simulink model "AFE_RC_OpenLoop"  (R2013b)
settings: Solver=FixedStepDiscrete  SolverMode=SingleTasking  StartTime=0.0  StopTime=5  FixedStep=Tpas  RelTol=1e-3
InitFcn:
  |  AFEsimpleparaDT1
values from neighbouring files (symbols this model uses):
  Freq = 50    [AFEsimpleparaDT1.m]
  hys = 100    [AFEsimpleparaDT1.m]
  Imax = 1.4697e+03    (= 1469.7)    [AFEsimpleparaDT1.m]
  Lac = 8.1487e-04    (= 0.00081487)    [AFEsimpleparaDT1.m]
  Tpas = 5e-5    (= 5e-05)    [AFEsimpleparaDT1.m]
  Vac = 2000    [AFEsimpleparaDT1.m]
libraries: powerlib x22, powerlib_meascontrol x7, simulink x6
settings Model: Creator=LiberT  LastModifiedBy=LiberT
settings DataIOCC: SignalLoggingSaveFormat=ModelDataLogs
settings OptimizationCC: ExpressionDepthLimit=2147483647
settings DebuggingCC: MultiTaskDSMMsg=warning  MultiTaskCondExecSysMsg=none  FcnCallInpInsideContextMsg=EnableAllAsWarning  StateNameClashWarn=warning
settings RTWCC: IncludeERTFirstTime=on

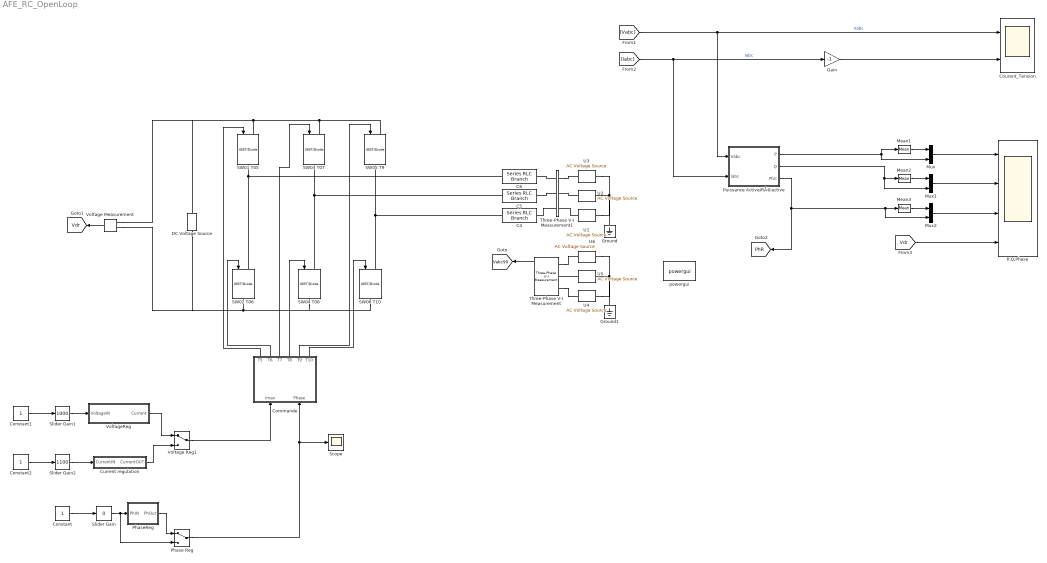
== system AFE_RC_OpenLoop ==
  C4 : powerlib/Elements/Series RLC Branch  LConnTagsString=__new0  RConnTagsString=__new0  BranchType=L  Resistance=(Vac*sqrt(2/3))^2  Inductance=Lac  SetiL0=off  InitialCurrent=0  Capacitance=300e-3  Setx0=off  InitialVoltage=0  Measurements=None
  C5 : powerlib/Elements/Series RLC Branch  LConnTagsString=__new0  RConnTagsString=__new0  BranchType=L  Resistance=(Vac*sqrt(2/3))^2  Inductance=Lac  SetiL0=off  InitialCurrent=0  Capacitance=300e-3  Setx0=off  InitialVoltage=0  Measurements=None
  C6 : powerlib/Elements/Series RLC Branch  LConnTagsString=__new0  RConnTagsString=__new0  BranchType=L  Resistance=(Vac*sqrt(2/3))^2  Inductance=Lac  SetiL0=off  InitialCurrent=0  Capacitance=300e-3  Setx0=off  InitialVoltage=0  Measurements=None
  Commande : Subsystem
  Constant : Constant
  Constant1 : Constant
  Constant2 : Constant
  Courant_Tension : Scope  NumInputPorts=2
      settings: TickLabels=on  TimeRange=0.04  YMin=-1750~-1750  YMax=1750~1750  SaveName=Courant_Tension  MaxDataPoints=50000
  Current regulation : Subsystem
  DC Voltage Source : powerlib/Electrical Sources/DC Voltage Source  Amplitude=5000  Measurements=None
  Gain : Gain  Gain=-1
  Ground : powerlib/Elements/Ground  LConnTagsString=a
  Ground1 : powerlib/Elements/Ground  LConnTagsString=a
  Mean1 : powerlib_meascontrol/Measurements/Mean  Freq=50  Vinit=0  Ts=Tpas
  Mean2 : powerlib_meascontrol/Measurements/Mean  Freq=50  Vinit=0  Ts=Tpas
  Mean3 : powerlib_meascontrol/Measurements/Mean  Freq=50  Vinit=0  Ts=Tpas
  Mux : Mux  Inputs=2
  Mux1 : Mux  Inputs=2
  Mux2 : Mux  Inputs=2
  P,Q,Phase : Scope  NumInputPorts=4
      settings: TickLabels=on  TimeRange=5  YMin=1.75e+06~-1.25e+06~-30~5000  YMax=4.5e+06~1.5e+06~25~5000  SaveName=PQ_Phi  MaxDataPoints=50000
  Phase Reg : ManualSwitch
  PhaseReg : Subsystem
  Puissance Active/RÃ©active : Subsystem
  SW01 T05 : powerlib/Power Electronics/IGBT//Diode  Ron=1e-3  Rs=1e5  Cs=Tpas  Measurements=off
  SW02 T06 : powerlib/Power Electronics/IGBT//Diode  Ron=1e-3  Rs=1e5  Cs=Tpas  Measurements=off
  SW03 T07 : powerlib/Power Electronics/IGBT//Diode  Ron=1e-3  Rs=1e5  Cs=Tpas  Measurements=off
  SW04 T08 : powerlib/Power Electronics/IGBT//Diode  Ron=1e-3  Rs=1e5  Cs=Tpas  Measurements=off
  SW05 T9 : powerlib/Power Electronics/IGBT//Diode  Ron=1e-3  Rs=1e5  Cs=Tpas  Measurements=off
  SW06 T10 : powerlib/Power Electronics/IGBT//Diode  Ron=1e-3  Rs=1e5  Cs=Tpas  Measurements=off
  Scope : Scope
      settings: YMin=-230  YMax=-160
  Slider Gain : simulink/Math Operations/Slider Gain  low=-180  gain=0  high=180
  Slider Gain1 : simulink/Math Operations/Slider Gain  low=0  gain=1000  high=5000
  Slider Gain2 : simulink/Math Operations/Slider Gain  low=500  gain=1100  high=1500
  Three-Phase V-I Measurement : powerlib/Measurements/Three-Phase V-I Measurement  VoltageMeasurement=phase-to-ground  SetLabelV=off  LabelV=Vabc  Vpu=off  VpuLL=off  CurrentMeasurement=no  SetLabelI=off  LabelI=Iabc  Ipu=off  Pbase=100e6  Vbase=500e3  OutputType=Complex  PhasorSimulation=off  PSBequivalent=0
  Three-Phase V-I Measurement1 : powerlib/Measurements/Three-Phase V-I Measurement  VoltageMeasurement=phase-to-ground  SetLabelV=on  LabelV=Vabc  Vpu=off  VpuLL=off  CurrentMeasurement=yes  SetLabelI=on  LabelI=Iabc  Ipu=off  Pbase=100e6  Vbase=500e3  OutputType=Complex  PhasorSimulation=off  PSBequivalent=0
  U1 : powerlib/Electrical Sources/AC Voltage Source  Amplitude=Vac*sqrt(2/3)  Phase=120  Frequency=Freq  SampleTime=Tpas  Measurements=Voltage
  U2 : powerlib/Electrical Sources/AC Voltage Source  Amplitude=Vac*sqrt(2/3)  Phase=-120  Frequency=Freq  SampleTime=Tpas  Measurements=Voltage
  U3 : powerlib/Electrical Sources/AC Voltage Source  Amplitude=Vac*sqrt(2/3)  Phase=0  Frequency=Freq  SampleTime=Tpas  Measurements=Voltage
  U4 : powerlib/Electrical Sources/AC Voltage Source  Amplitude=1  Phase=120-90  Frequency=Freq  SampleTime=Tpas  Measurements=Voltage
  U5 : powerlib/Electrical Sources/AC Voltage Source  Amplitude=1  Phase=-120-90  Frequency=Freq  SampleTime=Tpas  Measurements=Voltage
  U6 : powerlib/Electrical Sources/AC Voltage Source  Amplitude=1  Phase=-90  Frequency=Freq  SampleTime=Tpas  Measurements=Voltage
  Voltage Measurement : powerlib/Measurements/Voltage Measurement  PhasorSimulation=off  OutputType=Complex  PSBequivalent=0
  Voltage Reg1 : ManualSwitch
  VoltageReg : Subsystem
  powergui : powerlib/powergui  Priority=1  SimulationMode=Discrete  SolverType=Tustin  SampleTime=Tpas  frequency=50  SPID=off  DisableSnubberDevices=off  DisableRonSwitches=off  DisableVfSwitches=off  SwTol=0  Interpol=off  DisplayEquations=off  frequencyindice=50  Pbase=100e6  ErrMax=1e-4  Iterations=50  UnitsV=kV  UnitsW=MW  FunctionMessages=off  echomessages=off  HookPort=off  EnableUseOfTLC=off  x0status=blocks  RestoreLinks=warning  ResistiveCurrentMeasurement=off  Frange=[0:2:500]  Ylog=off  Xlog=on  ShowGrid=off  save=off  variable=ZData  structure=Courant_Tension  ZoomFFT=off  StartTime=0.5  cycles=225  DisplayStyle=1  fundamental=50  FreqAxis=off  MaxFrequency=500  frequencyindicesteady=1  RmsSteady=1  display=off  Ts=0  methode=off
  tag scope: PhR=global, Vabc90=global, Vdr=global
  wires:
  [Iabc] -> Gain/1, Puissance Active/RÃ©active/2(Iabc)  "Iabc"
  Commande/1(T5) -> SW01 T05/1
  Commande/2(T6) -> SW02 T06/1
  Commande/4(T8) -> SW04 T08/1
  Commande/3(T7) -> SW03 T07/1
  Commande/6(T10) -> SW06 T10/1
  Commande/5(T9) -> SW05 T9/1
  [Vabc] -> Courant_Tension/1, Puissance Active/RÃ©active/1(Vabc)  "Vabc"
  Voltage Measurement/1 -> [Vdr]
  [Vdr] -> P,Q,Phase/4
  Gain/1 -> Courant_Tension/2
  Three-Phase V-I Measurement/1 -> [Vabc90]
  Puissance Active/RÃ©active/3(PhC) -> [PhR], Mux2/2, Mean3/1
  Mux2/1 -> P,Q,Phase/3
  Puissance Active/RÃ©active/1(P) -> Mean1/1, Mux/2
  Mean1/1 -> Mux/1
  Mux/1 -> P,Q,Phase/1
  Mux1/1 -> P,Q,Phase/2
  Puissance Active/RÃ©active/2(Q) -> Mux1/2, Mean2/1
  Mean2/1 -> Mux1/1
  Mean3/1 -> Mux2/1
  Constant/1 -> Slider Gain/1
  Slider Gain/1 -> Phase Reg/2, PhaseReg/1(PhIN)
  PhaseReg/1(PhOut) -> Phase Reg/1
  Phase Reg/1 -> Commande/2(Phase), Scope/1
  Constant1/1 -> Slider Gain1/1
  Slider Gain1/1 -> VoltageReg/1(VoltageIN)
  Constant2/1 -> Slider Gain2/1
  Slider Gain2/1 -> Current regulation/1(CurrentIN)
  VoltageReg/1(Current) -> Voltage Reg1/1
  Current regulation/1(CurrentOUT) -> Voltage Reg1/2
  Voltage Reg1/1 -> Commande/1(Imax)
  connections:
  SW06 T10/RConn1 -- SW04 T08/RConn1 -- DC Voltage Source/LConn1 -- Voltage Measurement/LConn2 -- SW02 T06/RConn1
  SW01 T05/LConn1 -- DC Voltage Source/RConn1 -- Voltage Measurement/LConn1 -- SW05 T9/LConn1 -- SW03 T07/LConn1
  SW02 T06/LConn1 -- C6/LConn1 -- SW01 T05/RConn1
  SW06 T10/LConn1 -- C4/LConn1 -- SW05 T9/RConn1
  SW04 T08/LConn1 -- C5/LConn1 -- SW03 T07/RConn1
  U2/LConn1 -- U1/LConn1 -- Ground/LConn1 -- U3/LConn1
  Three-Phase V-I Measurement1/LConn1 -- C6/RConn1
  Three-Phase V-I Measurement1/RConn1 -- U3/RConn1
  U2/RConn1 -- Three-Phase V-I Measurement1/RConn2
  Three-Phase V-I Measurement1/LConn2 -- C5/RConn1
  C4/RConn1 -- Three-Phase V-I Measurement1/LConn3
  U1/RConn1 -- Three-Phase V-I Measurement1/RConn3
  U6/LConn1 -- U5/LConn1 -- U4/LConn1 -- Ground1/LConn1
  Three-Phase V-I Measurement/LConn1 -- U6/RConn1
  U5/RConn1 -- Three-Phase V-I Measurement/LConn2
  Three-Phase V-I Measurement/LConn3 -- U4/RConn1

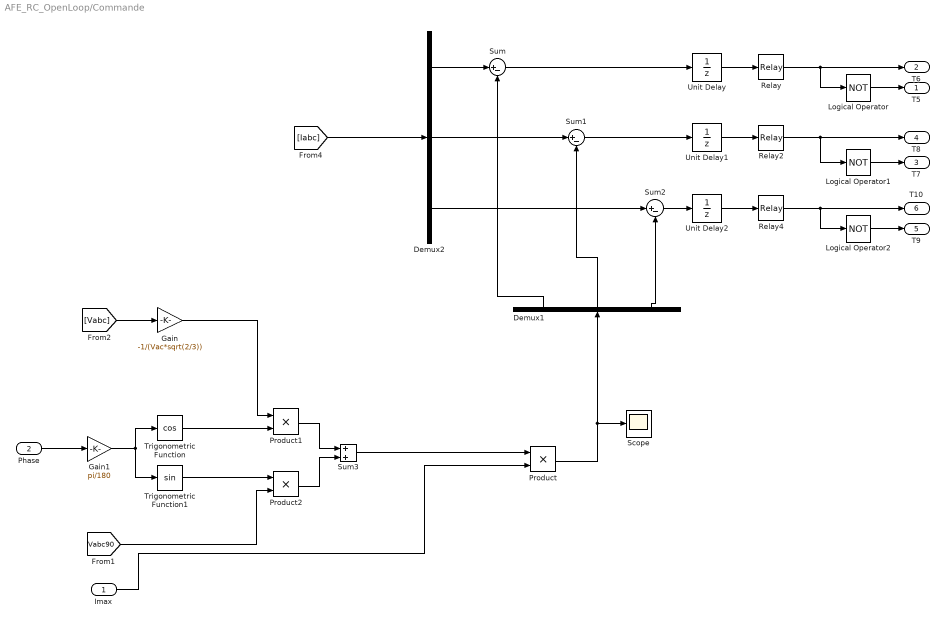
== system AFE_RC_OpenLoop/Commande ==
  Imax : Inport
  Phase : Inport  Port=2
  Demux1 : Demux  Outputs=3
  Demux2 : Demux  Outputs=3
  Gain : Gain  Gain=-1/(Vac*sqrt(2/3))
  Gain1 : Gain  Gain=pi/180
  Logical Operator : Logic  Operator=NOT  AllPortsSameDT=off
  Logical Operator1 : Logic  Operator=NOT  AllPortsSameDT=off
  Logical Operator2 : Logic  Operator=NOT  AllPortsSameDT=off
  Product : Product
  Product1 : Product
  Product2 : Product
  Relay : Relay  OnSwitchValue=hys  OffSwitchValue=-hys
  Relay2 : Relay  OnSwitchValue=hys  OffSwitchValue=-hys
  Relay4 : Relay  OnSwitchValue=hys  OffSwitchValue=-hys
  Scope : Scope
      settings: TimeRange=0.04  YMin=-1500  YMax=1500  MaxDataPoints=50000
  Sum : Sum  Inputs=|+-
  Sum1 : Sum  Inputs=|+-
  Sum2 : Sum  Inputs=|+-
  Sum3 : Sum
  Trigonometric Function : Trigonometry  Operator=cos
  Trigonometric Function1 : Trigonometry
  Unit Delay : UnitDelay  SampleTime=-1
  Unit Delay1 : UnitDelay  SampleTime=-1
  Unit Delay2 : UnitDelay  SampleTime=-1
  T5 : Outport
  T6 : Outport  Port=2
  T7 : Outport  Port=3
  T8 : Outport  Port=4
  T9 : Outport  Port=5
  T10 : Outport  Port=6
  wires:
  Demux2/1 -> Sum/1
  Demux2/2 -> Sum1/1
  Demux2/3 -> Sum2/1
  Sum/1 -> Unit Delay/1
  Sum1/1 -> Unit Delay1/1
  Sum2/1 -> Unit Delay2/1
  Unit Delay/1 -> Relay/1
  Unit Delay1/1 -> Relay2/1
  Unit Delay2/1 -> Relay4/1
  Logical Operator/1 -> T5/1
  Logical Operator1/1 -> T7/1
  Logical Operator2/1 -> T9/1
  Relay/1 -> T6/1, Logical Operator/1
  Relay2/1 -> T8/1, Logical Operator1/1
  Relay4/1 -> T10/1, Logical Operator2/1
  [Iabc] -> Demux2/1
  Demux1/2 -> Sum1/2
  Demux1/3 -> Sum2/2
  Demux1/1 -> Sum/2
  [Vabc] -> Gain/1
  Product/1 -> Scope/1, Demux1/1
  Gain/1 -> Product1/1
  Trigonometric Function/1 -> Product1/2
  [Vabc90] -> Product2/2
  Trigonometric Function1/1 -> Product2/1
  Product1/1 -> Sum3/1
  Product2/1 -> Sum3/2
  Sum3/1 -> Product/1
  Imax/1 -> Product/2
  Gain1/1 -> Trigonometric Function/1, Trigonometric Function1/1
  Phase/1 -> Gain1/1

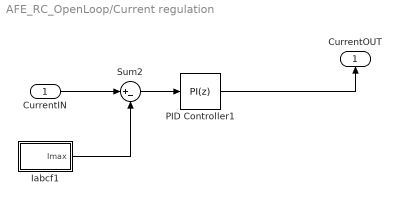
== system AFE_RC_OpenLoop/Current regulation ==
  CurrentIN : Inport
  Iabcf1 : Subsystem
  PID Controller1 : simulink/Continuous/PID Controller  Controller=PI  TimeDomain=Discrete-time  SampleTime=Tpas  IntegratorMethod=Forward Euler  FilterMethod=Forward Euler  Form=Parallel  P=5  I=0.1  D=0  N=100  InitialConditionSource=internal  InitialConditionForIntegrator=0  InitialConditionForFilter=0  ExternalReset=none  LimitOutput=on  UpperSaturationLimit=Imax  LowerSaturationLimit=0  LinearizeAsGain=on  AntiWindupMode=clamping  Kb=1  TrackingMode=off  Kt=1  PParamMin=[]  PParamMax=[]  IParamMin=[]  IParamMax=[]  DParamMin=[]  DParamMax=[]  NParamMin=[]  NParamMax=[]  KbParamMin=[]  KbParamMax=[]  KtParamMin=[]  KtParamMax=[]  POutMin=[]  POutMax=[]  IOutMin=[]  IOutMax=[]  DOutMin=[]  DOutMax=[]  NOutMin=[]  NOutMax=[]  KbOutMin=[]  KbOutMax=[]  KtOutMin=[]  KtOutMax=[]  IntegratorOutMin=[]  IntegratorOutMax=[]  FilterOutMin=[]  FilterOutMax=[]  SumOutMin=[]  SumOutMax=[]  SumI1OutMin=[]  SumI1OutMax=[]  SumI2OutMin=[]  SumI2OutMax=[]  SumI3OutMin=[]  SumI3OutMax=[]  SumDOutMin=[]  SumDOutMax=[]  SaturationOutMin=[]  SaturationOutMax=[]  IntegratorContinuousStateAttributes=''  IntegratorStateMustResolveToSignalObject=off  IntegratorRTWStateStorageClass=Auto  FilterContinuousStateAttributes=''  FilterStateMustResolveToSignalObject=off  FilterRTWStateStorageClass=Auto
  Sum2 : Sum  Inputs=|+-
  CurrentOUT : Outport
  wires:
  Iabcf1/1(Imax) -> Sum2/2
  PID Controller1/1 -> CurrentOUT/1
  Sum2/1 -> PID Controller1/1
  CurrentIN/1 -> Sum2/1

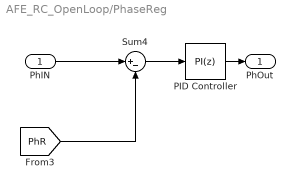
== system AFE_RC_OpenLoop/PhaseReg ==
  PhIN : Inport
  PID Controller : simulink/Continuous/PID Controller  Controller=PI  TimeDomain=Discrete-time  SampleTime=Tpas  IntegratorMethod=Forward Euler  FilterMethod=Forward Euler  Form=Parallel  P=0.48  I=8  D=0  N=100  InitialConditionSource=internal  InitialConditionForIntegrator=0  InitialConditionForFilter=0  ExternalReset=none  LimitOutput=off  UpperSaturationLimit=179.5  LowerSaturationLimit=-179.5  LinearizeAsGain=on  AntiWindupMode=clamping  Kb=1  TrackingMode=off  Kt=1  PParamMin=[]  PParamMax=[]  IParamMin=[]  IParamMax=[]  DParamMin=[]  DParamMax=[]  NParamMin=[]  NParamMax=[]  KbParamMin=[]  KbParamMax=[]  KtParamMin=[]  KtParamMax=[]  POutMin=[]  POutMax=[]  IOutMin=[]  IOutMax=[]  DOutMin=[]  DOutMax=[]  NOutMin=[]  NOutMax=[]  KbOutMin=[]  KbOutMax=[]  KtOutMin=[]  KtOutMax=[]  IntegratorOutMin=[]  IntegratorOutMax=[]  FilterOutMin=[]  FilterOutMax=[]  SumOutMin=[]  SumOutMax=[]  SumI1OutMin=[]  SumI1OutMax=[]  SumI2OutMin=[]  SumI2OutMax=[]  SumI3OutMin=[]  SumI3OutMax=[]  SumDOutMin=[]  SumDOutMax=[]  SaturationOutMin=[]  SaturationOutMax=[]  IntegratorContinuousStateAttributes=''  IntegratorStateMustResolveToSignalObject=off  IntegratorRTWStateStorageClass=Auto  FilterContinuousStateAttributes=''  FilterStateMustResolveToSignalObject=off  FilterRTWStateStorageClass=Auto
  Sum4 : Sum  Inputs=|+-
  PhOut : Outport
  wires:
  PID Controller/1 -> PhOut/1
  Sum4/1 -> PID Controller/1
  [PhR] -> Sum4/2
  PhIN/1 -> Sum4/1

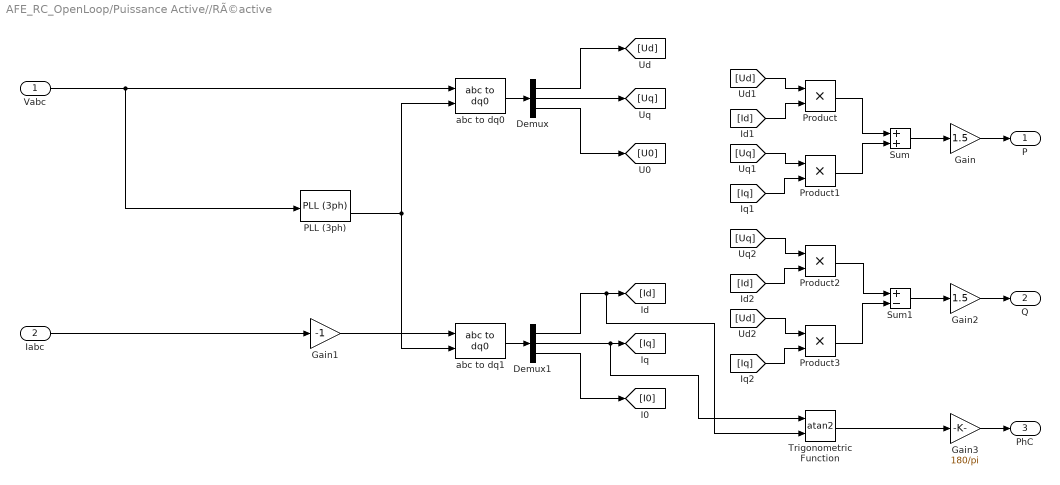
== system AFE_RC_OpenLoop/Puissance Active//RÃ©active ==
  Vabc : Inport
  Iabc : Inport  Port=2
  Demux : Demux  Outputs=3
  Demux1 : Demux  Outputs=3
  Gain : Gain  Gain=1.5
  Gain1 : Gain  Gain=-1
  Gain2 : Gain  Gain=1.5
  Gain3 : Gain  Gain=180/pi
  PLL (3ph) : powerlib_meascontrol/PLL/PLL (3ph)  Fmin=49  Par_Init=[0, 50]  ParK=[180, 3200, 1]  TcD=1e-4  MaxRateChangeFreq=6  FilterCutOffFreq=25  Ts=Tpas  AGC=on
  Product{,1..3} (4 alike) : Product
  Sum : Sum
  Sum1 : Sum  Inputs=+-
  Trigonometric Function : Trigonometry  Operator=atan2
  abc to dq0 : powerlib_meascontrol/Transformations/abc to dq0  Alignment=90 degrees behind phase A axis
  abc to dq1 : powerlib_meascontrol/Transformations/abc to dq0  Alignment=90 degrees behind phase A axis
  P : Outport
  Q : Outport  Port=2
  PhC : Outport  Port=3
  wires:
  Vabc/1 -> PLL (3ph)/1, abc to dq0/1
  abc to dq0/1 -> Demux/1
  abc to dq1/1 -> Demux1/1
  Product/1 -> Sum/1
  Product3/1 -> Sum1/2
  PLL (3ph)/2 -> abc to dq0/2, abc to dq1/2
  Sum1/1 -> Gain2/1
  Sum/1 -> Gain/1
  Demux/1 -> [Ud]
  Demux/2 -> [Uq]
  Demux/3 -> [U0]
  Demux1/1 -> Trigonometric Function/2, [Id]
  Demux1/2 -> Trigonometric Function/1, [Iq]
  Demux1/3 -> [I0]
  [Ud] -> Product/1
  [Id] -> Product/2
  [Uq] -> Product1/1
  [Iq] -> Product1/2
  [Uq] -> Product2/1
  [Id] -> Product2/2
  [Ud] -> Product3/1
  [Iq] -> Product3/2
  Product1/1 -> Sum/2
  Gain1/1 -> abc to dq1/1
  Product2/1 -> Sum1/1
  Gain/1 -> P/1
  Gain2/1 -> Q/1
  Iabc/1 -> Gain1/1
  Trigonometric Function/1 -> Gain3/1
  Gain3/1 -> PhC/1

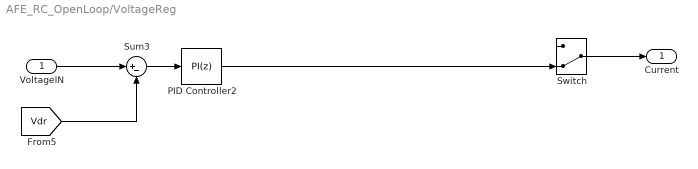
== system AFE_RC_OpenLoop/VoltageReg ==
  VoltageIN : Inport
  " Switch" : ManualSwitch  CurrentSetting=0
  PID Controller2 : simulink/Continuous/PID Controller  Controller=PI  TimeDomain=Discrete-time  SampleTime=Tpas  IntegratorMethod=Forward Euler  FilterMethod=Forward Euler  Form=Parallel  P=5  I=20  D=0  N=100  InitialConditionSource=internal  InitialConditionForIntegrator=0  InitialConditionForFilter=0  ExternalReset=none  LimitOutput=on  UpperSaturationLimit=1000  LowerSaturationLimit=-1000  LinearizeAsGain=on  AntiWindupMode=clamping  Kb=1  TrackingMode=off  Kt=1  PParamMin=[]  PParamMax=[]  IParamMin=[]  IParamMax=[]  DParamMin=[]  DParamMax=[]  NParamMin=[]  NParamMax=[]  KbParamMin=[]  KbParamMax=[]  KtParamMin=[]  KtParamMax=[]  POutMin=[]  POutMax=[]  IOutMin=[]  IOutMax=[]  DOutMin=[]  DOutMax=[]  NOutMin=[]  NOutMax=[]  KbOutMin=[]  KbOutMax=[]  KtOutMin=[]  KtOutMax=[]  IntegratorOutMin=[]  IntegratorOutMax=[]  FilterOutMin=[]  FilterOutMax=[]  SumOutMin=[]  SumOutMax=[]  SumI1OutMin=[]  SumI1OutMax=[]  SumI2OutMin=[]  SumI2OutMax=[]  SumI3OutMin=[]  SumI3OutMax=[]  SumDOutMin=[]  SumDOutMax=[]  SaturationOutMin=[]  SaturationOutMax=[]  IntegratorContinuousStateAttributes=''  IntegratorStateMustResolveToSignalObject=off  IntegratorRTWStateStorageClass=Auto  FilterContinuousStateAttributes=''  FilterStateMustResolveToSignalObject=off  FilterRTWStateStorageClass=Auto
  Sum3 : Sum  Inputs=|+-
  Current : Outport
  wires:
  Sum3/1 -> PID Controller2/1
  VoltageIN/1 -> Sum3/1
  [Vdr] -> Sum3/2
  " Switch"/1 -> Current/1
  PID Controller2/1 -> " Switch"/2

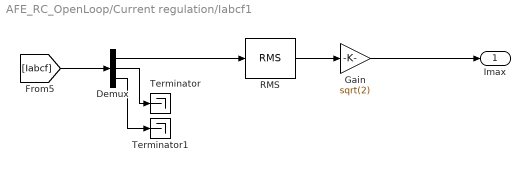
== system AFE_RC_OpenLoop/Current regulation/Iabcf1 ==
  Demux : Demux  Outputs=3
  Gain : Gain  Gain=sqrt(2)  SampleTime=Tpas
  RMS : powerlib_meascontrol/Measurements/RMS  TrueRMS=on  Freq=Freq  RMSInit=0  Ts=Tpas
  Terminator : Terminator
  Terminator1 : Terminator
  Imax : Outport
  wires:
  [Iabcf] -> Demux/1
  Demux/3 -> Terminator1/1
  Demux/2 -> Terminator/1
  Demux/1 -> RMS/1
  RMS/1 -> Gain/1
  Gain/1 -> Imax/1
